simulink model "Task_1_SC_model"  (R2020a)
settings: Solver=VariableStepAuto  StartTime=0.0  StopTime=1000  MaxStep=1e-3  RelTol=1e-3
values from neighbouring files (symbols this model uses):
  I_r = 0.005    [Input_data_Task1.m]
  I_x = 0.07    [Input_data_Task1.m]
  I_y = 0.0504    [Input_data_Task1.m]
  I_z = 0.0109    [Input_data_Task1.m]
settings Model: Creator=dvdia  LastModifiedBy=dvdia

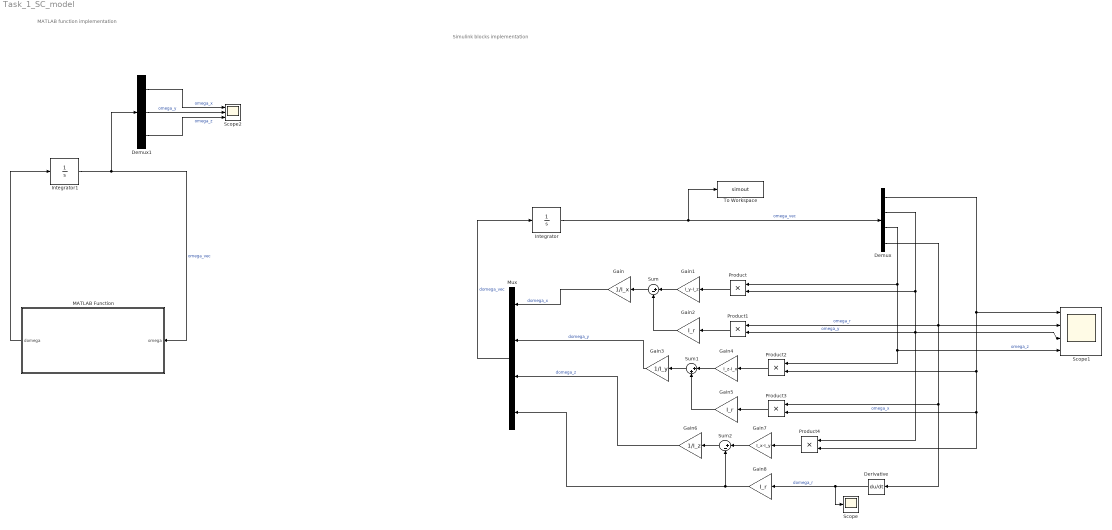
== system Task_1_SC_model ==
  note: MATLAB function implementation
  note: Simulink blocks implementation
  Demux : Demux
  Demux1 : Demux  Outputs=3
  Derivative : Derivative
  Gain : Gain  Gain=1/I_x
  Gain1 : Gain  Gain=I_y-I_z
  Gain2 : Gain  Gain=I_r
  Gain3 : Gain  Gain=1/I_y
  Gain4 : Gain  Gain=I_z-I_x
  Gain5 : Gain  Gain=I_r
  Gain6 : Gain  Gain=1/I_z
  Gain7 : Gain  Gain=I_x-I_y
  Gain8 : Gain  Gain=I_r
  Integrator : Integrator  InitialCondition=[1.e-6 1.e-6 0.02 2*pi]
  Integrator1 : Integrator  InitialCondition=[1.e-6 1.e-6 0.02]
  MATLAB Function : MATLAB Function  TreatAsAtomicUnit=on
  Mux : Mux
  Product{,1..4} (5 alike) : Product
  Scope : Scope
  Scope1 : Scope  NumInputPorts=4
  Scope2 : Scope  NumInputPorts=3
  Sum : Sum  Inputs=|+-
  Sum1 : Sum  Inputs=|++
  Sum2 : Sum  Inputs=|+-
  To Workspace : ToWorkspace  VariableName=simout  SampleTime=-1
  wires:
  Gain/1 -> Mux/1  "domega_x"
  Sum/1 -> Gain/1
  Gain1/1 -> Sum/1
  Product/1 -> Gain1/1
  Gain2/1 -> Sum/2
  Product1/1 -> Gain2/1
  Demux/4 -> Scope1/2, Product3/1, Derivative/1, Product1/1  "omega_r"
  Mux/1 -> Integrator/1  "domega_vec"
  Product3/1 -> Gain5/1
  Gain5/1 -> Sum1/2
  Demux/3 -> Product2/1, Scope1/4, Product/1  "omega_z"
  Product2/1 -> Gain4/1
  Gain4/1 -> Sum1/1
  Sum1/1 -> Gain3/1
  Gain3/1 -> Mux/2  "domega_y"
  Integrator/1 -> To Workspace/1, Demux/1  "omega_vec"
  Gain6/1 -> Mux/3  "domega_z"
  Sum2/1 -> Gain6/1
  Gain7/1 -> Sum2/1
  Product4/1 -> Gain7/1
  Demux/2 -> Product/2, Product4/1, Scope1/3, Product1/2  "omega_y"
  Demux/1 -> Product2/2, Product3/2, Product4/2, Scope1/1  "omega_x"
  Gain8/1 -> Mux/4, Sum2/2
  Derivative/1 -> Scope/1, Gain8/1  "domega_r"
  MATLAB Function/1(domega) -> Integrator1/1
  Integrator1/1 -> Demux1/1, MATLAB Function/1(omega)  "omega_vec"
  Demux1/1 -> Scope2/1  "omega_x"
  Demux1/2 -> Scope2/2  "omega_y"
  Demux1/3 -> Scope2/3  "omega_z"

== matlab function Task_1_SC_model/MATLAB Function ==
  data: omega input; domega output
function domega = fcn(omega)

% Inertia moments

I_x = 0.07;         %  [kg*m^2]
I_y = 0.0504;       %  [kg*m^2]
I_z = 0.0109;       %  [kg*m^2]
I_r = 0.005;        %  [kg*m^2]

% Initial conditions

omega0_vec = [1.e-6 1.e-6 0.02 2*pi];

% Set omegas
omega_x = omega(1);
omega_y = omega(2);
omega_z = omega(3);
omega_r = 2*pi;         % omega_r is constant

% Compute d_omegas
domega_x = ((I_y-I_z)*omega_y*omega_z - I_r * omega_r * omega_y)/I_x;
domega_y = ((I_z-I_x)*omega_x*omega_z + I_r * omega_r * omega_x)/I_y;
domega_z = (I_x - I_y)*omega_y*omega_x / I_z;
domega = [ domega_x domega_y domega_z ];
end
